simulink model "zad2model2"  (R2023a)
settings: Solver=VariableStepAuto  StartTime=0.0  StopTime=30  RelTol=1e-3
values from neighbouring files (symbols this model uses):
  Gz = c2d(Gs,T,'zoh')    [zad1.m]
  T = 0.5    [zad1.m]    (also in zad4.mat)
settings Model: Creator=pkutyl  LastModifiedBy=pkutyl

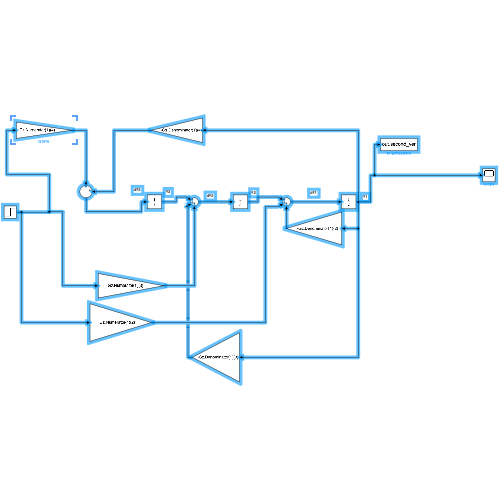
[thumbnail: Simulink's stored preview of the top-level diagram]
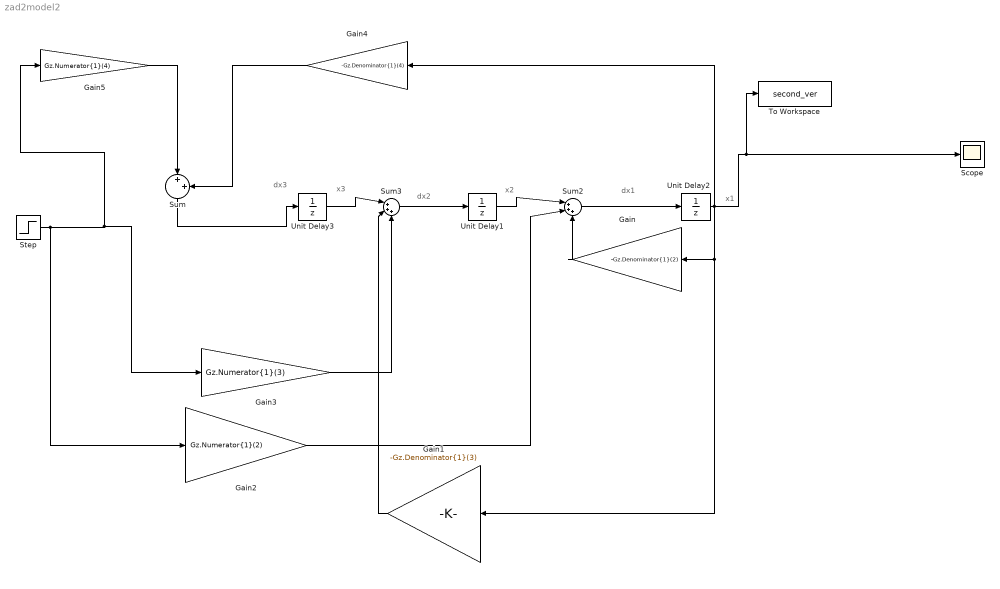
== system zad2model2 ==
  note: dx3
  note: x3
  note: dx2
  note: x2
  note: dx1
  note: x1
  Gain : Gain  Gain=-Gz.Denominator{1}(2)
  Gain1 : Gain  Gain=-Gz.Denominator{1}(3)
  Gain2 : Gain  Gain=Gz.Numerator{1}(2)
  Gain3 : Gain  Gain=Gz.Numerator{1}(3)
  Gain4 : Gain  Gain=-Gz.Denominator{1}(4)
  Gain5 : Gain  Gain=Gz.Numerator{1}(4)
  Scope : Scope
  Step : Step  Time=0  SampleTime=T
  Sum : Sum  Inputs=|++
  Sum2 : Sum  Inputs=|+++
  Sum3 : Sum  Inputs=|+++
  To Workspace : ToWorkspace  VariableName=second_ver  SaveFormat=Structure With Time  SampleTime=-1
  Unit Delay1 : UnitDelay  SampleTime=T  HasFrameUpgradeWarning=on
  Unit Delay2 : UnitDelay  SampleTime=T  HasFrameUpgradeWarning=on
  Unit Delay3 : UnitDelay  SampleTime=T  HasFrameUpgradeWarning=on
  wires:
  Unit Delay2/1 -> Gain1/1, Gain/1, To Workspace/1, Scope/1, Gain4/1
  Step/1 -> Gain3/1, Gain5/1, Gain2/1
  Sum/1 -> Unit Delay3/1
  Unit Delay1/1 -> Sum2/1
  Sum2/1 -> Unit Delay2/1
  Unit Delay3/1 -> Sum3/1
  Sum3/1 -> Unit Delay1/1
  Gain1/1 -> Sum3/2
  Gain2/1 -> Sum2/2
  Gain3/1 -> Sum3/3
  Gain4/1 -> Sum/2
  Gain5/1 -> Sum/1
  Gain/1 -> Sum2/3
